simulink model "robot_velocities"  (R2019b)
settings: Solver=VariableStepAuto  StartTime=0.0  StopTime=inf  RelTol=1e-3
values from neighbouring files (symbols this model uses):
  sampleTime = 0.1    [main.m]
libraries: mobileRoboticsLib x4
settings Model: EnablePacing=on  Creator=adityaaaap  LastModifiedBy=adityaaaap

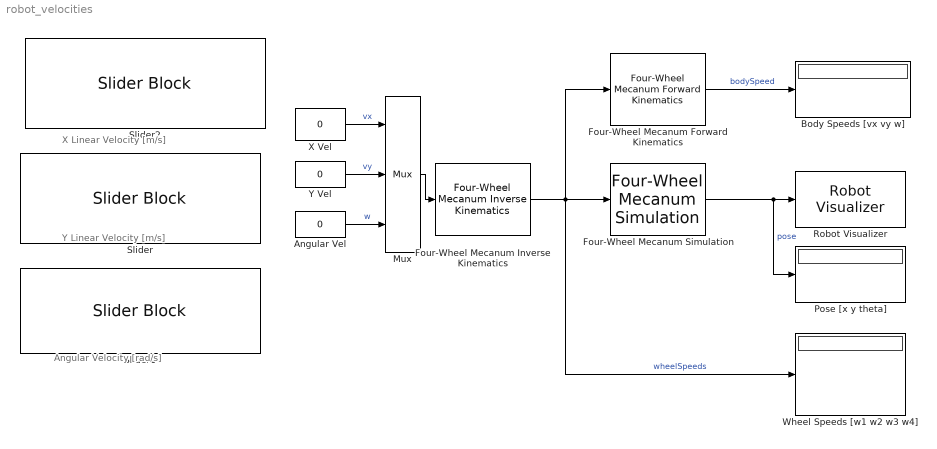
== system robot_velocities ==
  note: X Linear Velocity [m/s]
  note: Y Linear Velocity [m/s]
  note: Angular Velocity [rad/s]
  Angular Vel : Constant  Value=0
  Body Speeds [vx vy w] : Display
  Four-Wheel Mecanum Forward Kinematics : mobileRoboticsLib/Kinematic Models/Four-Wheel Mecanum/Four-Wheel Mecanum Forward Kinematics  wheelRadius=wheelRadius  wheelBase=wheelBase  wheelTrack=wheelTrack
      settings: SourceProductName=Mobile Robotics Simulation Library
  Four-Wheel Mecanum Inverse Kinematics : mobileRoboticsLib/Kinematic Models/Four-Wheel Mecanum/Four-Wheel Mecanum Inverse Kinematics  wheelRadius=wheelRadius  wheelBase=wheelBase  wheelTrack=wheelTrack
      settings: SourceProductName=Mobile Robotics Simulation Library
  Four-Wheel Mecanum Simulation : mobileRoboticsLib/Kinematic Models/Four-Wheel Mecanum/Four-Wheel Mecanum Simulation  wheelRadius=wheelRadius  wheelBase=wheelBase  wheelTrack=wheelTrack  initX=0  initY=0  initAngle=0  Ts=sampleTime
      settings: SourceProductName=Mobile Robotics Simulation Library
  Mux : Mux  Inputs=3
  Pose [x y theta] : Display
  Robot Visualizer : mobileRoboticsLib/Environments/Robot Visualizer  Priority=99  robotRadius=0  showTrajectory=on  hasWaypoints=off  hasLidar=off  sensorOffset=[ 0 0 ]  scanAngles=scanAngles  hasObjDetector=off  objDetectorOffset=[ 0, 0 ]  objDetectorAngle=0  objDetectorFOV=pi/4  objDetectorMaxRange=5  objectColors=[ 1, 0, 0; 0, 1, 0; 0, 0, 1 ]  objectMarkers=s
      settings: SourceProductName=Ground Vehicles Library
  Slider : SliderBlock  ScaleMin=-1  ScaleMax=1  TickInterval=0.25
  Slider1 : SliderBlock  ScaleMin=-1.5  ScaleMax=1.5
  Slider2 : SliderBlock  ScaleMin=-1  ScaleMax=1  TickInterval=0.25
  Wheel Speeds [w1 w2 w3 w4] : Display
  X Vel : Constant  Value=0
  Y Vel : Constant  Value=0
  wires:
  Four-Wheel Mecanum Forward Kinematics/1 -> Body Speeds [vx vy w]/1  "bodySpeed"
  Angular Vel/1 -> Mux/3  "w"
  X Vel/1 -> Mux/1  "vx"
  Mux/1 -> Four-Wheel Mecanum Inverse Kinematics/1
  Four-Wheel Mecanum Inverse Kinematics/1 -> Four-Wheel Mecanum Forward Kinematics/1, Four-Wheel Mecanum Simulation/1, Wheel Speeds [w1 w2 w3 w4]/1  "wheelSpeeds"
  Four-Wheel Mecanum Simulation/1 -> Pose [x y theta]/1, Robot Visualizer/1  "pose"
  Y Vel/1 -> Mux/2  "vy"
